simulink model "c1_chirp_filter"  (R2020b)
settings: Solver=FixedStepDiscrete  StartTime=0.0  StopTime=stopTime  FixedStep=2.0833333333333333e-05  RelTol=1e-3
values from neighbouring files (symbols this model uses):
  cihc = 1    [modelparameters.m]
  norm_gainc1 = (sqrt(C1gain_norm))/((sqrt(CF^2+rzero^2))^order_of_zero)    [c1_chirp_parameter.m]    (also in modelparameters.m)
settings Model: Creator=Ross  LastModifiedBy=conno
settings DataIOCC: SaveOutput=off  SaveTime=off  ReturnWorkspaceOutputs=off
settings OptimizationCC: BlockReduction=off  ConditionallyExecuteInputs=off  DefaultParameterBehavior=Inlined
settings DebuggingCC: ReadBeforeWriteMsg=DisableAll  WriteAfterWriteMsg=DisableAll  WriteAfterReadMsg=DisableAll  AlgebraicLoopMsg=error  MultiTaskDSMMsg=none  SingleTaskRateTransMsg=error  PregeneratedLibrarySubsystemCodeDiagnostic=none  ArithmeticOperatorsInVariantConditions=warning
settings HardwareCC: ProdBitPerPointer=32  ProdBitPerSizeT=32  ProdBitPerPtrDiffT=32  ProdLargestAtomicFloat=None  ProdIntDivRoundTo=Undefined  ProdEndianess=Unspecified  ProdWordSize=32  ProdHWDeviceType=ASIC/FPGA->ASIC/FPGA  TargetBitPerPointer=64  TargetBitPerSizeT=64  TargetBitPerPtrDiffT=64  TargetLongLongMode=on  TargetIntDivRoundTo=Zero  TargetEndianess=LittleEndian  TargetWordSize=64  TargetHWDeviceType=Custom Processor->MATLAB Host Computer  ProdEqTarget=off
settings ModelReferenceCC: UpdateModelReferenceTargets=IfOutOfDate  ModelReferenceNumInstancesAllowed=Single
settings SFSimCC: SFSimEcho=off  SimUseLocalCustomCode=off  CustomCodeUndefinedFunction=UseInterfaceOnly
settings RTWCC: RTWUseLocalCustomCode=off

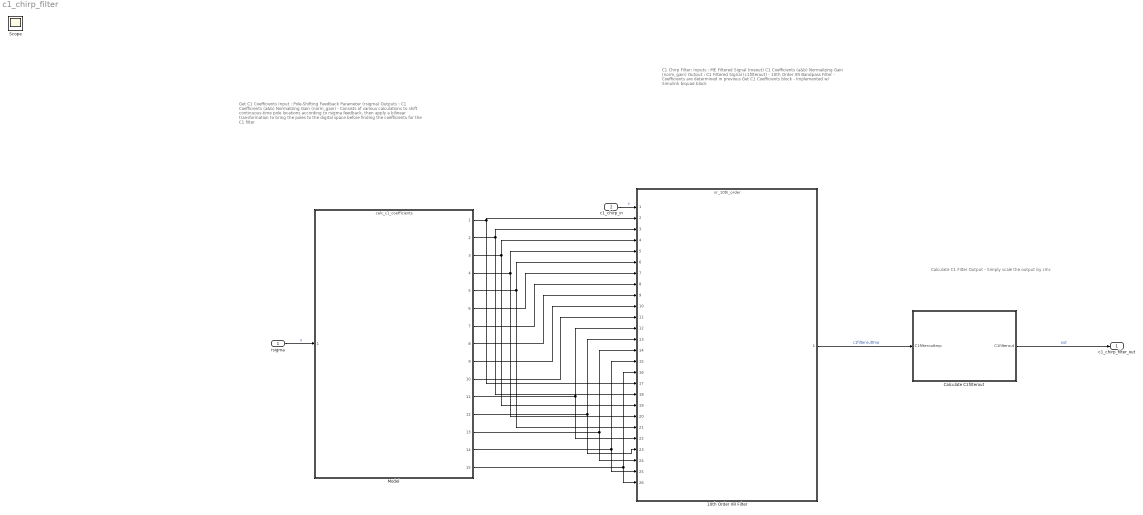
== system c1_chirp_filter ==
  note: Calculate C1 Filter Output
      |
      | - Simply scale the output by cihc
  note: Get C1 Coefficients
      |
      | Input : Pole-Shifting Feedback Parameter (rsigma)
      |
      | Outputs : C1 Coefficients (a&b)
      | Normalizing Gain (norm_gain)
      |
      | - Consists of various calculations to shift continuous-time pole locations according to rsigma feedback, then apply a bilinear transformation to bring the poles to the digital space before finding the coefficients for the C1 filter
  note: C1 Chirp Filter:
      |
      | Inputs : ME Filtered Signal (meout)
      | C1 Coefficients (a&b)
      | Normalizing Gain (norm_gain)
      |
      | Output : C1 Filtered Signal (c1filterout)
      |
      | - 10th Order IIR Bandpass Filter
      |
      | - Coefficients are determined in previous Get C1 Coefficients block
      |
      | - Implemented w/ Simulink biquad block
  rsigma : Inport  OutDataTypeStr=single  PortDimensions=1  SampleTime=[2.0833333333333333e-05,0]
  c1_chirp_in : Inport  Port=2  OutDataTypeStr=single  PortDimensions=1  SampleTime=[2.0833333333333333e-05,0]
  10th Order IIR Filter : ModelReference  ModelNameDialog=iir_10th_order  SimulationMode=Normal  ModelReferenceVersion=1.114
  Calculate C1filterout : Subsystem
  Model : ModelReference  ModelNameDialog=calc_c1_coefficients.slx  SimulationMode=Normal  ModelReferenceVersion=1.150
  c1_chirp_filter_out : Outport  OutDataTypeStr=single  PortDimensions=1  SampleTime=[2.0833333333333333e-05,0]  VectorParamsAs1DForOutWhenUnconnected=off
  Scope : Scope
  wires:
  10th Order IIR Filter/1 -> Calculate C1filterout/1(C1filterouttmp)  "c1filterouttmp"
  rsigma/1 -> Model/1  "x"
  c1_chirp_in/1 -> 10th Order IIR Filter/1  "x"
  Calculate C1filterout/1(C1filterout) -> c1_chirp_filter_out/1  "out"
  Model/1 -> 10th Order IIR Filter/2, 10th Order IIR Filter/17
  Model/2 -> 10th Order IIR Filter/3, 10th Order IIR Filter/18
  Model/3 -> 10th Order IIR Filter/19, 10th Order IIR Filter/4
  Model/4 -> 10th Order IIR Filter/20, 10th Order IIR Filter/5
  Model/5 -> 10th Order IIR Filter/21, 10th Order IIR Filter/6
  Model/6 -> 10th Order IIR Filter/7
  Model/7 -> 10th Order IIR Filter/8
  Model/8 -> 10th Order IIR Filter/9
  Model/9 -> 10th Order IIR Filter/10
  Model/10 -> 10th Order IIR Filter/11
  Model/11 -> 10th Order IIR Filter/22, 10th Order IIR Filter/12
  Model/12 -> 10th Order IIR Filter/13, 10th Order IIR Filter/23
  Model/13 -> 10th Order IIR Filter/24, 10th Order IIR Filter/14
  Model/14 -> 10th Order IIR Filter/25, 10th Order IIR Filter/15
  Model/15 -> 10th Order IIR Filter/26, 10th Order IIR Filter/16

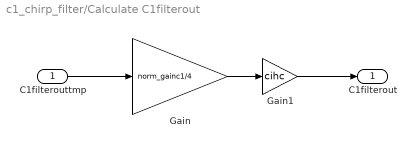
== system c1_chirp_filter/Calculate C1filterout ==
  C1filterouttmp : Inport
  Gain : Gain  Gain=norm_gainc1/4
  Gain1 : Gain  Gain=cihc
  C1filterout : Outport  VectorParamsAs1DForOutWhenUnconnected=off
  wires:
  Gain1/1 -> C1filterout/1
  Gain/1 -> Gain1/1
  C1filterouttmp/1 -> Gain/1
